simulink model "nlmpc_ZonePcm_RBC"  (R2020b)
settings: Solver=VariableStepAuto  StartTime=0.0  StopTime=86400*2  RelTol=1e-6
settings Model: Creator=taoy  LastModifiedBy=taoy
settings SolverCC: AlgebraicLoopSolver=LineSearch

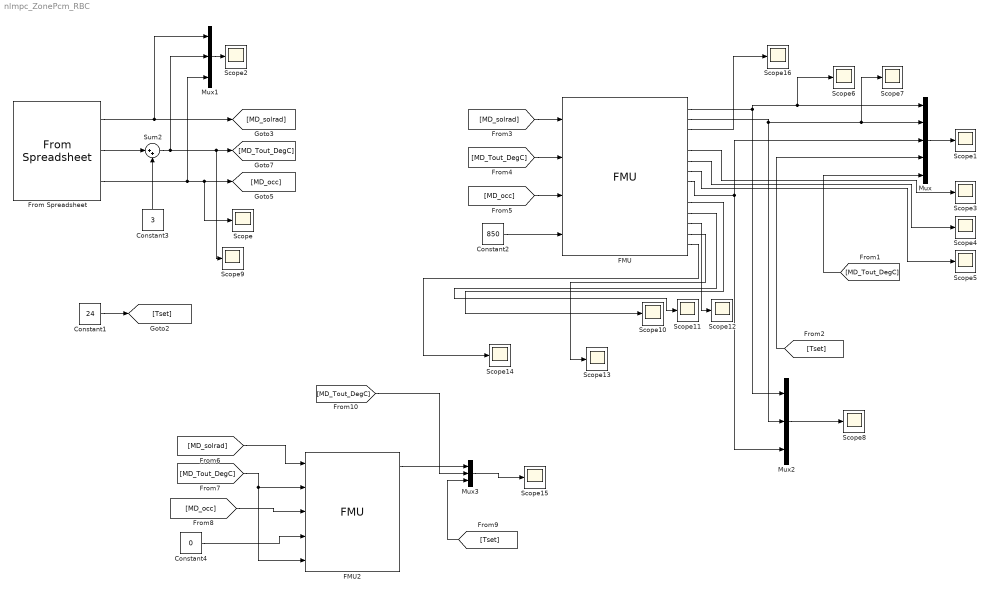
== system nlmpc_ZonePcm_RBC ==
  Constant1 : Constant  Value=24  SampleTime=Inf
  Constant2 : Constant  Value=850  SampleTime=Inf
  Constant3 : Constant  Value=3  SampleTime=Inf
  Constant4 : Constant  Value=0  SampleTime=Inf
  FMU : FMU  FMUName=RBC_10_new.fmu  FMUMode=CoSimulation  system=struct('p_ambient',101325,'T_ambient',293.15,'g',9.80665,'m_flow_start',0,'eps_m_flow',0.0001,'dp_small',1,'m_flow_small',0.01)  TairInit=20  mPC_demo4_1=struct('TAirInit_2',20,'CO2Init',400,'RExt',2.0,'RInt',0.05,'tmass',25,'imass',17.89,'shgc',1.985,'CO2n',400,'CO2pp',0.039,'maxVent',1746,'vent',1746,'occ_gain',20.0,'maxHeat',1310,'prescribedHeatFlow',struct('T_ref',293.15,'alpha',0),'occHeatGain',struct('T_ref',293.15,'alpha',0),'Vi',121.625,'occheff',1.0,'Vinf',50,'airMix_new',struct('h_to_s',struct('k',0.0002777777777777778),'AirRhoCp',struct('k',1206.0),'multiProduct',struct('significantDigits',int32(8)),'prescribedHeatFlow',struct('T_ref',293.15,'alpha',0),'add1',struct('k1',1,'k2',-1)),'integrator',struct('k',1,'y_start',0),'Tve',21)  aHU_PCM_one_stack_NoData=struct('PCM1',struct('Tinit',22.0,'heatCapacitor',struct('cp_s',2000,'cp_l',2000,'hf_pcm',140000,'m_pcm',1),'convection_coefficient1',struct('m_PCM_2',100,'k_a',0.02364,'rho_a',1.288,'my_a',1.729E-05,'Pr_a',0.7344,'L_CSM',0.45,'H_c',0.0015,'Nu_rest',7.54),'thermalConductor',struct('G_2',15),'Area',struct('k',0.135),'Lf',struct('Bh',2.118,'Bc',18.37,'Tmc',294.71,'Tmh',295.46999999999997,'vh',2.804,'vc',31.11)),'rho',struct('k',1.288),'boundary',struct('X',[0.01,0.99],'m_flow',0,'T',293.15),'gain1',struct('k',0.0002777777777777778),'gain2',struct('k',0.010416666666666666),'bou',struct('X',[0.01,0.99],'p',101325,'h',45300.945),'vol',struct('p_start',101325,'T_start',293.15,'X_start',[0.01,0.99],'m_flow_nominal',0.0036,'V',0.00010125000000000001))  add=struct('k1',-1,'k2',1)  cp=struct('k',0.00036908333333333335)  multiProduct=struct('significantDigits',int32(3))  const=struct('k',0)  const1=struct('k',0)  const2=struct('k',24)  gain=struct('k',96)  gain1=struct('k',3600)  zeroOrderHold=struct('samplePeriod',60,'startTime',0)  zeroOrderHold1=struct('samplePeriod',60,'startTime',0)  zeroOrderHold2=struct('samplePeriod',60,'startTime',0)  mask(RBC_10_new [Co-Simulation, v2.0]){}
      mask Display:
      | disp('RBC_10_new');
      | port_label('output',1,'Tin');
      | port_label('output',2,'Tsup');
      | port_label('output',3,'H');
      | port_label('output',4,'dHdT');
      | port_label('output',5,'Qc');
      | port_label('output',6,'qc');
      | port_label('output',7,'Qsup');
      | port_label('output',8,'Tpcm');
      | port_label('output',9,'Tinterior');
      | port_label('output',10,'y1');
      | port_label('output',11,'y2');
      | port_label('output',12,'y3');
      | port_label('output',13,'Vair_out');
      | port_label('output',14,'k');
      | port_label('input',1,'solrad');
      | port_label('input',2,'Tout');
      | port_label('input',3,'occ');
      | port_label('input',4,'Vair');
  FMU2 : FMU  FMUName=zone_3.fmu  FMUMode=CoSimulation  TAirInit=20  CO2Init=400  RExt=2  RInt=0.05  tmass=25  imass=17.89  shgc=1.985  CO2n=400  CO2pp=0.039  maxVent=1746  vent=1746  occ_gain=25.0  maxHeat=1310  prescribedHeatFlow=struct('T_ref',293.15,'alpha',0)  occHeatGain=struct('T_ref',293.15,'alpha',0)  Vi=486.5/4  occheff=1.0  Vinf=50  airMix_new=struct('h_to_s',struct('k',0.0002777777777777778),'AirRhoCp',struct('k',1206.0),'multiProduct',struct('significantDigits',int32(8)),'prescribedHeatFlow',struct('T_ref',293.15,'alpha',0),'add1',struct('k1',1,'k2',-1))  integrator=struct('k',1,'y_start',0)  Tve=21  mask(zone_3 [Co-Simulation, v2.0]){}
      mask Display:
      | disp('zone_3');
      | port_label('output',1,'Tin');
      | port_label('output',2,'Qrad');
      | port_label('output',3,'qrad');
      | port_label('output',4,'Tinterior');
      | port_label('input',1,'Solrad');
      | port_label('input',2,'Tout');
      | port_label('input',3,'Occ');
      | port_label('input',4,'Vair');
      | port_label('input',5,'Tsup');
  From Spreadsheet : FromSpreadsheet  FileName=meas_q.csv  SheetName=meas_q  SampleTime=900
  Mux : Mux  Inputs=5
  Mux1 : Mux  Inputs=3
  Mux2 : Mux  Inputs=3
  Mux3 : Mux  Inputs=3
  Scope{,1..16} (17 alike) : Scope
  Sum2 : Sum  Inputs=|++
  wires:
  From Spreadsheet/1 -> Mux1/1, [MD_solrad]
  [MD_solrad] -> FMU/1
  From Spreadsheet/2 -> Sum2/1
  Sum2/1 -> Mux1/2, Scope9/1, [MD_Tout_DegC]
  Constant3/1 -> Sum2/2
  [MD_Tout_DegC] -> FMU/2
  [Tset] -> Mux/4
  [MD_Tout_DegC] -> Mux/5
  Mux/1 -> Scope1/1
  Mux1/1 -> Scope2/1
  Constant1/1 -> [Tset]
  Constant2/1 -> FMU/4
  FMU/1 -> Scope6/1, Mux/1, Mux2/1
  FMU/2 -> Mux2/2, Scope7/1, Mux/2
  FMU/5 -> Scope3/1
  FMU/6 -> Scope4/1
  FMU/7 -> Scope5/1
  FMU/8 -> Mux2/3, Mux/3
  Mux2/1 -> Scope8/1
  FMU/10 -> Scope10/1
  FMU/11 -> Scope11/1
  FMU/12 -> Scope12/1
  FMU/13 -> Scope13/1
  [MD_occ] -> FMU/3
  From Spreadsheet/3 -> Mux1/3, Scope/1, [MD_occ]
  FMU/14 -> Scope14/1
  [MD_solrad] -> FMU2/1
  [MD_Tout_DegC] -> FMU2/5, FMU2/2
  [MD_Tout_DegC] -> Mux3/2
  [Tset] -> Mux3/3
  [MD_occ] -> FMU2/3
  Constant4/1 -> FMU2/4
  FMU2/1 -> Mux3/1
  Mux3/1 -> Scope15/1
  FMU/3 -> Scope16/1
